simulink model "SimpleImpedanceControl"  (R2019b)
settings: Solver=VariableStepAuto  StartTime=0.0  StopTime=100  FixedStep=0.001  RelTol=10^-6
model workspace: external: MATLAB File /home/sydney/Desktop/matlab/simulink/SimpImpCheck/Assembly1_DataFile.m (data not in the file)
undefined symbols (not defined in the file or in its folder): smiData, X, Y, Z
libraries: sm_lib x21, fl_lib x17, nesl_utility x17, ee_lib x3
(part 2 of 2)

== matlab function SimpleImpedanceControl/MATLAB Function2 ==
  data: var1 input; outputArray output; var2 input; var3 input
function outputArray = collate(var1, var2, var3)

outputArray = [var1,var2,var3];
